simulink model "FromPeripherals"  (R2016b)
settings: Solver=VariableStepAuto  StartTime=0.0  StopTime=10.0  RelTol=1e-3
settings Model: Creator=Nathan  LastModifiedBy=Nathan

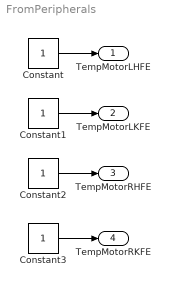
== system FromPeripherals ==
  Constant{,1..3} (4 alike) : Constant
  TempMotorLHFE : Outport
  TempMotorLKFE : Outport  Port=2
  TempMotorRHFE : Outport  Port=3
  TempMotorRKFE : Outport  Port=4
  wires:
  Constant/1 -> TempMotorLHFE/1
  Constant1/1 -> TempMotorLKFE/1
  Constant2/1 -> TempMotorRHFE/1
  Constant3/1 -> TempMotorRKFE/1
